simulink model "viperModel_NoFingers"  (R2022a)
settings: Solver=VariableStepAuto  StartTime=0.0  StopTime=10.0  RelTol=1e-3
undefined symbols (not defined in the file or in its folder): smiData, X, Y, Z
libraries: nesl_utility x186, sm_lib x71
(part 3 of 3)

== system viperModel_NoFingers/vx300_wrist_link1 ==
  Inertia : sm_lib/Body Elements/Inertia  InertiaType=Custom  Mass=0.115395  MassUnits=kg  CenterOfMass=[0, 0, 0]  CenterOfMassUnits=m  MomentsOfInertia=[4.631e-05, 4.514e-05, 5.27e-05]  MomentsOfInertiaUnits=kg*m^2  ProductsOfInertia=[4.2002e-06, 2.3e-09, 1.95e-08]  ProductsOfInertiaUnits=kg*m^2  GraphicType=None  MarkerShape=Inertia  MarkerSize=20  GraphicVisPropType=SimpleVisualProperties  GraphicDiffuseColor=[0.5 0.5 0.5]  GraphicSpecularColor=[0.5 0.5 0.5 1.0]  GraphicAmbientColor=[0.15 0.15 0.15 1.0]  GraphicEmissiveColor=[0.0 0.0 0.0 1.0]  GraphicShininess=75  GraphicOpacity=1.0
  InertiaOriginTransform : sm_lib/Frames and Transforms/Rigid Transform  TranslationMethod=Cartesian  TranslationStandardOffset=0  TranslationLengthUnit=m  TranslationStandardAxis=+Z  TranslationCartesianOffset=[0.046743, -7.665200000000001e-06, 0.010565]  TranslationROffset=0  TranslationROffsetUnits=m  TranslationZOffset=0  TranslationZOffsetUnits=m  TranslationThetaOffset=0  TranslationThetaOffsetUnits=deg  RotationMethod=RotationSequence  RotationAngleUnits=deg  RotationStandardAxis=+Z  RotationAngle=0.0  RotationArbitraryAxis=[0 0 1]  FollAlignAxisA=+X  BaseAlignAxisA=+Y  FollAlignAxisB=+Y  BaseAlignAxisB=+Z  RotationSequenceAxes=BaseAxes  RotationSequence=XYZ  RotationSequenceAngles=[0, 0, 1.570796326794897]  RotationSequenceAnglesUnits=rad  RotationMatrix=[1 0 0; 0 1 0; 0 0 1]
  ReferenceFrame : sm_lib/Frames and Transforms/Reference Frame
  Visual : sm_lib/Body Elements/File Solid  ExtGeomFileName=ViperX_300/interbotix_xsarm_descriptions/meshes/vx300_meshes/vx300_5_wrist.stl  UnitType=Custom  ExtGeomFileUnits=mm  StepReaderType=HEX  ExportConvexHullGeometry=off  InertiaType=Custom  Mass=0  MassUnits=kg  CenterOfMass=[0, 0, 0]  CenterOfMassUnits=m  MomentsOfInertia=[0, 0, 0]  MomentsOfInertiaUnits=kg*m^2  ProductsOfInertia=[0, 0, 0]  ProductsOfInertiaUnits=kg*m^2  BasedOnType=DensityFromFile  Density=1000  DensityUnits=kg/m^3  DoExposeReferenceFrame=on  SerializedFrames=<Frames/>  GraphicType=FromGeometry  MarkerShape=Sphere  MarkerSize=10  GraphicVisPropType=SimpleVisualProperties  GraphicDiffuseColor=[0.5, 0.5, 0.5]  GraphicSpecularColor=[0.5 0.5 0.5 1.0]  GraphicAmbientColor=[0.15 0.15 0.15 1.0]  GraphicEmissiveColor=[0.0 0.0 0.0 1.0]  GraphicShininess=75  GraphicOpacity=1
  VisualOriginTransform : sm_lib/Frames and Transforms/Rigid Transform  TranslationMethod=Cartesian  TranslationStandardOffset=0  TranslationLengthUnit=m  TranslationStandardAxis=+Z  TranslationCartesianOffset=[0, 0, 0]  TranslationROffset=0  TranslationROffsetUnits=m  TranslationZOffset=0  TranslationZOffsetUnits=m  TranslationThetaOffset=0  TranslationThetaOffsetUnits=deg  RotationMethod=RotationSequence  RotationAngleUnits=deg  RotationStandardAxis=+Z  RotationAngle=0.0  RotationArbitraryAxis=[0 0 1]  FollAlignAxisA=+X  BaseAlignAxisA=+Y  FollAlignAxisB=+Y  BaseAlignAxisB=+Z  RotationSequenceAxes=BaseAxes  RotationSequence=XYZ  RotationSequenceAngles=[0, 0, 1.570796326794897]  RotationSequenceAnglesUnits=rad  RotationMatrix=[1 0 0; 0 1 0; 0 0 1]
  wrist_angle_AxisInvTransform : sm_lib/Frames and Transforms/Rigid Transform  TranslationMethod=Cartesian  TranslationStandardOffset=0  TranslationLengthUnit=m  TranslationStandardAxis=+Z  TranslationCartesianOffset=[0, 0, 0]  TranslationROffset=0  TranslationROffsetUnits=m  TranslationZOffset=0  TranslationZOffsetUnits=m  TranslationThetaOffset=0  TranslationThetaOffsetUnits=deg  RotationMethod=ArbitraryAxis  RotationAngleUnits=rad  RotationStandardAxis=+Z  RotationAngle=1.570796326794897  RotationArbitraryAxis=[-1, 0, 0]  FollAlignAxisA=+X  BaseAlignAxisA=+Y  FollAlignAxisB=+Y  BaseAlignAxisB=+Z  RotationSequenceAxes=FollowerAxes  RotationSequence=XYX  RotationSequenceAngles=[0 0 0]  RotationSequenceAnglesUnits=deg  RotationMatrix=[1 0 0; 0 1 0; 0 0 1]
  wrist_rotate_AxisTransform : sm_lib/Frames and Transforms/Rigid Transform  TranslationMethod=Cartesian  TranslationStandardOffset=0  TranslationLengthUnit=m  TranslationStandardAxis=+Z  TranslationCartesianOffset=[0, 0, 0]  TranslationROffset=0  TranslationROffsetUnits=m  TranslationZOffset=0  TranslationZOffsetUnits=m  TranslationThetaOffset=0  TranslationThetaOffsetUnits=deg  RotationMethod=ArbitraryAxis  RotationAngleUnits=rad  RotationStandardAxis=+Z  RotationAngle=1.570796326794897  RotationArbitraryAxis=[-0, 1, 0]  FollAlignAxisA=+X  BaseAlignAxisA=+Y  FollAlignAxisB=+Y  BaseAlignAxisB=+Z  RotationSequenceAxes=FollowerAxes  RotationSequence=XYX  RotationSequenceAngles=[0 0 0]  RotationSequenceAnglesUnits=deg  RotationMatrix=[1 0 0; 0 1 0; 0 0 1]
  wrist_rotate_OriginTransform : sm_lib/Frames and Transforms/Rigid Transform  TranslationMethod=Cartesian  TranslationStandardOffset=0  TranslationLengthUnit=m  TranslationStandardAxis=+Z  TranslationCartesianOffset=[0.069744, 0, 0]  TranslationROffset=0  TranslationROffsetUnits=m  TranslationZOffset=0  TranslationZOffsetUnits=m  TranslationThetaOffset=0  TranslationThetaOffsetUnits=deg  RotationMethod=RotationSequence  RotationAngleUnits=deg  RotationStandardAxis=+Z  RotationAngle=0.0  RotationArbitraryAxis=[0 0 1]  FollAlignAxisA=+X  BaseAlignAxisA=+Y  FollAlignAxisB=+Y  BaseAlignAxisB=+Z  RotationSequenceAxes=BaseAxes  RotationSequence=XYZ  RotationSequenceAngles=[0, 0, 0]  RotationSequenceAnglesUnits=rad  RotationMatrix=[1 0 0; 0 1 0; 0 0 1]
  F : PMIOPort  Side=Left
  F1 : PMIOPort  Port=2  Side=Right
  connections:
  wrist_rotate_AxisTransform/LConn1 -- wrist_rotate_OriginTransform/RConn1
  wrist_rotate_AxisTransform/RConn1 -- F1/RConn1
  wrist_angle_AxisInvTransform/RConn1 -- F/RConn1
  Visual/RConn1 -- VisualOriginTransform/RConn1
  VisualOriginTransform/LConn1 -- ReferenceFrame/RConn1 -- InertiaOriginTransform/LConn1 -- wrist_rotate_OriginTransform/LConn1 -- wrist_angle_AxisInvTransform/LConn1
  Inertia/RConn1 -- InertiaOriginTransform/RConn1

== matlab function viperModel_NoFingers/State_Output3/QuatToEuler321 ==
  data: q input; euler output
function euler  = callQuatToEuler321(q)


[euler] = quatToEuler_321(q);

== matlab function viperModel_NoFingers/State_Output3/formPoseMat ==
  data: rotMat input; mat output; posVec input
function mat  = callFormPoseMat(rotMat,posVec)


[mat] = formPoseMat(rotMat,posVec);

== matlab function viperModel_NoFingers/State_Output4/MATLAB Function ==
  data: qin input; qout output
function qout = call_quatconj(qin)

qout = zeros(1,4);
qout = quatconj(qin');

== matlab function viperModel_NoFingers/State_Output4/QuatToDCM ==
  data: q input; mat output
function mat  = callQuatToDCM(q)

[mat] = quatToDCM(q);

== matlab function viperModel_NoFingers/State_Output4/QuatToEuler321 ==
  data: q input; euler output
function euler  = callQuatToEuler321(q)


[euler] = quatToEuler_321(q);

== matlab function viperModel_NoFingers/State_Output4/formPoseMat ==
  data: rotMat input; mat output; posVec input
function mat  = callFormPoseMat(rotMat,posVec)


[mat] = formPoseMat(rotMat,posVec);

== matlab function viperModel_NoFingers/State_Output5/MATLAB Function ==
  data: qin input; qout output
function qout = call_quatconj(qin)

qout = zeros(1,4);
qout = quatconj(qin');

== matlab function viperModel_NoFingers/State_Output5/QuatToDCM ==
  data: q input; mat output
function mat  = callQuatToDCM(q)

[mat] = quatToDCM(q);

== matlab function viperModel_NoFingers/State_Output5/QuatToEuler321 ==
  data: q input; euler output
function euler  = callQuatToEuler321(q)


[euler] = quatToEuler_321(q);

== matlab function viperModel_NoFingers/State_Output5/formPoseMat ==
  data: rotMat input; mat output; posVec input
function mat  = callFormPoseMat(rotMat,posVec)


[mat] = formPoseMat(rotMat,posVec);

== matlab function viperModel_NoFingers/State_Output6/MATLAB Function ==
  data: qin input; qout output
function qout = call_quatconj(qin)

qout = zeros(1,4);
qout = quatconj(qin');

== matlab function viperModel_NoFingers/State_Output6/QuatToDCM ==
  data: q input; mat output
function mat  = callQuatToDCM(q)

[mat] = quatToDCM(q);

== matlab function viperModel_NoFingers/State_Output6/QuatToEuler321 ==
  data: q input; euler output
function euler  = callQuatToEuler321(q)


[euler] = quatToEuler_321(q);

== matlab function viperModel_NoFingers/State_Output6/formPoseMat ==
  data: rotMat input; mat output; posVec input
function mat  = callFormPoseMat(rotMat,posVec)


[mat] = formPoseMat(rotMat,posVec);

== matlab function viperModel_NoFingers/State_Output7/MATLAB Function ==
  data: qin input; qout output
function qout = call_quatconj(qin)

qout = zeros(1,4);
qout = quatconj(qin');

== matlab function viperModel_NoFingers/State_Output7/QuatToDCM ==
  data: q input; mat output
function mat  = callQuatToDCM(q)

[mat] = quatToDCM(q);

== matlab function viperModel_NoFingers/State_Output7/QuatToEuler321 ==
  data: q input; euler output
function euler  = callQuatToEuler321(q)


[euler] = quatToEuler_321(q);

== matlab function viperModel_NoFingers/State_Output7/formPoseMat ==
  data: rotMat input; mat output; posVec input
function mat  = callFormPoseMat(rotMat,posVec)


[mat] = formPoseMat(rotMat,posVec);

== matlab function viperModel_NoFingers/State_Output8/MATLAB Function ==
  data: qin input; qout output
function qout = call_quatconj(qin)

qout = zeros(1,4);
qout = quatconj(qin');

== matlab function viperModel_NoFingers/State_Output8/QuatToDCM ==
  data: q input; mat output
function mat  = callQuatToDCM(q)

[mat] = quatToDCM(q);

== matlab function viperModel_NoFingers/State_Output8/QuatToEuler321 ==
  data: q input; euler output
function euler  = callQuatToEuler321(q)


[euler] = quatToEuler_321(q);

== matlab function viperModel_NoFingers/State_Output8/formPoseMat ==
  data: rotMat input; mat output; posVec input
function mat  = callFormPoseMat(rotMat,posVec)


[mat] = formPoseMat(rotMat,posVec);

== matlab function viperModel_NoFingers/State_Output9/MATLAB Function ==
  data: qin input; qout output
function qout = call_quatconj(qin)

qout = zeros(1,4);
qout = quatconj(qin');

== matlab function viperModel_NoFingers/State_Output9/QuatToDCM ==
  data: q input; mat output
function mat  = callQuatToDCM(q)

[mat] = quatToDCM(q);

== matlab function viperModel_NoFingers/State_Output9/QuatToEuler321 ==
  data: q input; euler output
function euler  = callQuatToEuler321(q)


[euler] = quatToEuler_321(q);

== matlab function viperModel_NoFingers/State_Output9/formPoseMat ==
  data: rotMat input; mat output; posVec input
function mat  = callFormPoseMat(rotMat,posVec)


[mat] = formPoseMat(rotMat,posVec);

== matlab function viperModel_NoFingers/State_Output10/MATLAB Function ==
  data: qin input; qout output
function qout = call_quatconj(qin)

qout = zeros(1,4);
qout = quatconj(qin');

== matlab function viperModel_NoFingers/State_Output10/QuatToDCM ==
  data: q input; mat output
function mat  = callQuatToDCM(q)

[mat] = quatToDCM(q);

== matlab function viperModel_NoFingers/State_Output1/MATLAB Function ==
  data: qin input; qout output
function qout = call_quatconj(qin)

qout = zeros(1,4);
qout = quatconj(qin');

== matlab function viperModel_NoFingers/State_Output10/QuatToEuler321 ==
  data: q input; euler output
function euler  = callQuatToEuler321(q)


[euler] = quatToEuler_321(q);

== matlab function viperModel_NoFingers/State_Output10/formPoseMat ==
  data: rotMat input; mat output; posVec input
function mat  = callFormPoseMat(rotMat,posVec)


[mat] = formPoseMat(rotMat,posVec);

== matlab function viperModel_NoFingers/State_Output1/QuatToDCM ==
  data: q input; mat output
function mat  = callQuatToDCM(q)

[mat] = quatToDCM(q);

== matlab function viperModel_NoFingers/State_Output1/QuatToEuler321 ==
  data: q input; euler output
function euler  = callQuatToEuler321(q)


[euler] = quatToEuler_321(q);

== matlab function viperModel_NoFingers/State_Output1/formPoseMat ==
  data: rotMat input; mat output; posVec input
function mat  = callFormPoseMat(rotMat,posVec)


[mat] = formPoseMat(rotMat,posVec);

== matlab function viperModel_NoFingers/State_Output2/MATLAB Function ==
  data: qin input; qout output
function qout = call_quatconj(qin)

qout = zeros(1,4);
qout = quatconj(qin');

== matlab function viperModel_NoFingers/State_Output2/QuatToDCM ==
  data: q input; mat output
function mat  = callQuatToDCM(q)

[mat] = quatToDCM(q);

== matlab function viperModel_NoFingers/State_Output2/QuatToEuler321 ==
  data: q input; euler output
function euler  = callQuatToEuler321(q)


[euler] = quatToEuler_321(q);

== matlab function viperModel_NoFingers/State_Output2/formPoseMat ==
  data: rotMat input; mat output; posVec input
function mat  = callFormPoseMat(rotMat,posVec)


[mat] = formPoseMat(rotMat,posVec);

== matlab function viperModel_NoFingers/State_Output3/MATLAB Function ==
  data: qin input; qout output
function qout = call_quatconj(qin)

qout = zeros(1,4);
qout = quatconj(qin');

== matlab function viperModel_NoFingers/State_Output3/QuatToDCM ==
  data: q input; mat output
function mat  = callQuatToDCM(q)

[mat] = quatToDCM(q);
